simulink model "MRR_H8_Alap"  (R2025a)
settings: Solver=VariableStepAuto  StartTime=0.0  StopTime=20.0  MaxStep=1/25  RelTol=1e-3
InitFcn:
  | K = 1;
  | tau = 1;
  | xi = 1;
settings Model: Creator=Szalay  LastModifiedBy=Szalay

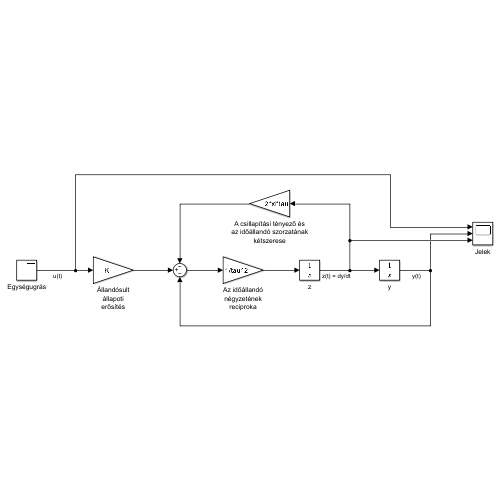
[thumbnail: Simulink's stored preview of the top-level diagram]
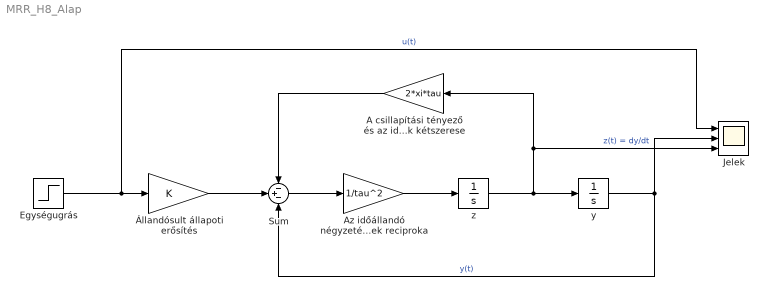
== system MRR_H8_Alap ==
  A csillapítási tényező és az időállandó szorzatának kétszerese : Gain  Gain=2*xi*tau
  Az időállandó négyzetének reciproka : Gain  Gain=1/tau^2
  Egységugrás : Step  SampleTime=0
  Jelek : Scope  NumInputPorts=3
      settings: ActiveDisplayYMinimum=-0.24557420987255357  ActiveDisplayYMaximum=1.3195316345107526
  Sum : Sum  Inputs=-+-
  y : Integrator
  z : Integrator
  Állandósult állapoti erősítés : Gain  Gain=K
  wires:
  z/1 -> Jelek/3, A csillapítási tényező és az időállandó szorzatának kétszerese/1, y/1  "z(t) = dy/dt"
  Az időállandó négyzetének reciproka/1 -> z/1
  Sum/1 -> Az időállandó négyzetének reciproka/1
  Állandósult állapoti erősítés/1 -> Sum/2
  A csillapítási tényező és az időállandó szorzatának kétszerese/1 -> Sum/1
  y/1 -> Jelek/2, Sum/3  "y(t)"
  Egységugrás/1 -> Jelek/1, Állandósult állapoti erősítés/1  "u(t)"
